simulink model "Model_8"  (R2020b)
settings: Solver=VariableStepAuto  StartTime=0.0  StopTime=10.0  RelTol=1e-3
settings Model: EnablePacing=on  PacingRate=0.100000  Creator=Akarsh  LastModifiedBy=Akarsh

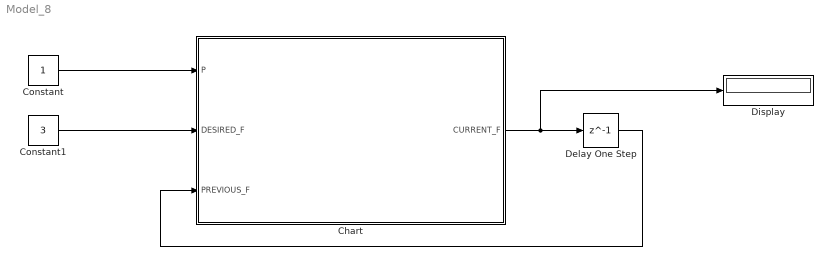
== system Model_8 ==
  Chart : Stateflow chart  TreatAsAtomicUnit=on
  Constant : Constant
  Constant1 : Constant  Value=3
  Delay One Step : Delay  DelayLength=1
  Display : Display
  wires:
  Chart/1(CURRENT_F) -> Display/1, Delay One Step/1
  Delay One Step/1 -> Chart/3(PREVIOUS_F)
  Constant/1 -> Chart/1(P)
  Constant1/1 -> Chart/2(DESIRED_F)

== stateflow chart Model_8/Chart ==
  state POWER_ON
  state MOVING_UP
    CURRENT_F=CURRENT_F+1
  state POWER_OFF
    CURRENT_F=PREVIOUS_F
  state MOVING_DOWN
    CURRENT_F=CURRENT_F-1
  MOVING_UP -> MOVING_UP [order 2] : [CURRENT_F~=DESIRED_F]
  POWER_ON -> MOVING_UP [order 3] : [DESIRED_F>CURRENT_F]
  POWER_OFF -> POWER_ON : [P==1]
  MOVING_UP -> POWER_OFF [order 1] : [CURRENT_F==DESIRED_F]
  POWER_ON -> POWER_OFF [order 1] : [P==0]
  POWER_ON -> MOVING_DOWN [order 2] : [DESIRED_F<CURRENT_F]
  (default) -> POWER_OFF
  MOVING_DOWN -> POWER_OFF [order 2] : [CURRENT_F==DESIRED_F]
  MOVING_DOWN -> MOVING_DOWN [order 1] : [CURRENT_F ~= DESIRED_F]
  data: P input; DESIRED_F input; CURRENT_F output; PREVIOUS_F input
